simulink model "drgania"  (Simulink 7.1)
settings: Solver=ode45  StartTime=0.0  StopTime=100  RelTol=1e-3
settings Model: Creator=surbaniak  LastModifiedBy=surbaniak

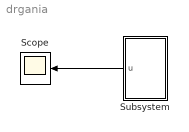
== system drgania ==
  Scope : Scope
  Subsystem : Subsystem  Orientation=left  mask{k1=80000, k2=500000, m2=320, m1=2500, b1=350, b2=15020}
  wires:
  Subsystem/1(u) -> Scope/1

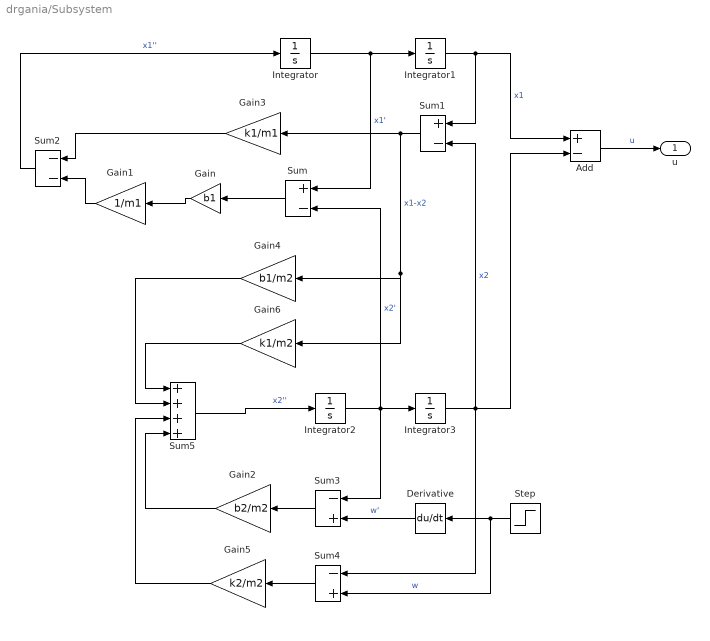
== system drgania/Subsystem ==
  Add : Sum  Inputs=+-  OutDataType=sfix(16)  OutScaling=2^-10
  Derivative : Derivative  Orientation=left
  Gain : Gain  Orientation=left  Gain=b1  ParameterDataType=sfix(16)  ParameterScaling=2^0  OutDataType=sfix(16)  OutScaling=2^0
  Gain1 : Gain  Orientation=left  Gain=1/m1  ParameterDataType=sfix(16)  ParameterScaling=2^0  OutDataType=sfix(16)  OutScaling=2^0
  Gain2 : Gain  Orientation=left  Gain=b2/m2  ParameterDataType=sfix(16)  ParameterScaling=2^0  OutDataType=sfix(16)  OutScaling=2^0
  Gain3 : Gain  Orientation=left  Gain=k1/m1  ParameterDataType=sfix(16)  ParameterScaling=2^0  OutDataType=sfix(16)  OutScaling=2^0
  Gain4 : Gain  Orientation=left  Gain=b1/m2  ParameterDataType=sfix(16)  ParameterScaling=2^0  OutDataType=sfix(16)  OutScaling=2^0
  Gain5 : Gain  Orientation=left  Gain=k2/m2  ParameterDataType=sfix(16)  ParameterScaling=2^0  OutDataType=sfix(16)  OutScaling=2^0
  Gain6 : Gain  Orientation=left  Gain=k1/m2  ParameterDataType=sfix(16)  ParameterScaling=2^0  OutDataType=sfix(16)  OutScaling=2^0
  Integrator{,1..3} (4 alike) : Integrator
  Step : Step  Orientation=left  After=0.01  SampleTime=0
  Sum : Sum  Orientation=left  Inputs=+-  OutDataType=sfix(16)  OutScaling=2^0
  Sum1 : Sum  Orientation=left  Inputs=+-  OutDataType=sfix(16)  OutScaling=2^0
  Sum2 : Sum  Orientation=left  Inputs=--  OutDataType=sfix(16)  OutScaling=2^0
  Sum3 : Sum  Orientation=left  Inputs=-+  OutDataType=sfix(16)  OutScaling=2^0
  Sum4 : Sum  Orientation=left  Inputs=-+  OutDataType=sfix(16)  OutScaling=2^0
  Sum5 : Sum  Inputs=++++  OutDataType=sfix(16)  OutScaling=2^0
  u : Outport  OutDataType=sfix(16)  OutScaling=2^0
  wires:
  Integrator/1 -> Integrator1/1, Sum/1  "x1'"
  Integrator2/1 -> Integrator3/1, Sum/2, Sum3/1  "x2'"
  Integrator1/1 -> Add/1, Sum1/1  "x1"
  Integrator3/1 -> Add/2, Sum1/2, Sum4/1  "x2"
  Sum/1 -> Gain/1
  Gain/1 -> Gain1/1
  Sum1/1 -> Gain3/1, Gain4/1, Gain6/1  "x1-x2"
  Gain3/1 -> Sum2/1
  Gain1/1 -> Sum2/2
  Sum2/1 -> Integrator/1  "x1''"
  Step/1 -> Derivative/1, Sum4/2  "w"
  Derivative/1 -> Sum3/2  "w'"
  Sum3/1 -> Gain2/1
  Sum4/1 -> Gain5/1
  Sum5/1 -> Integrator2/1  "x2''"
  Gain6/1 -> Sum5/1
  Gain4/1 -> Sum5/2
  Gain2/1 -> Sum5/4
  Gain5/1 -> Sum5/3
  Add/1 -> u/1  "u"
